simulink model "px4demo_Send_All_Data"  (R2016b)
settings: Solver=FixedStepDiscrete  StartTime=0.0  StopTime=inf  FixedStep=0.01  RelTol=1e-3  EnableMultiTasking=on
undefined symbols (not defined in the file): dt_pixhawk
libraries: pixhawk_slib_sensors_actuators x8, pixhawk_slib_ADC_serial x2
settings Model: Creator=darenlee  LastModifiedBy=ers
settings DataIOCC: LimitDataPoints=on  SaveFormat=StructureWithTime
settings OptimizationCC: DefaultParameterBehavior=Inlined  LifeSpan=1  MaxStackSize=64
settings DebuggingCC: AllowSymbolicDim=off  SFUnexpectedBacktrackingDiag=warning  SFNoUnconditionalDefaultTransitionDiag=warning  SFExecutionAtInitializationDiag=none
settings HardwareCC: ProdBitPerPointer=32  ProdBitPerSizeT=32  ProdBitPerPtrDiffT=32  ProdLargestAtomicInteger=Long  ProdLargestAtomicFloat=Double  ProdIntDivRoundTo=Undefined  ProdWordSize=32  ProdHWDeviceType=ARM Compatible->ARM Cortex
settings ModelReferenceCC: PropagateSignalLabelsOutOfModel=off
settings RTWCC: SystemTargetFile=ert.tlc  HardwareBoard=Pixhawk PX4  TLCOptions=-aInlineSetEventsForThisBaseRateFcn=TLC_FALSE -aSuppressMultiTaskScheduler=TLC_FALSE -aRateBasedStepFcn=0  TemplateMakefile=ert_default_tmf  Description=Embedded Coder  GenerateReport=on  Toolchain=Pixhawk Toolchain  IncludeHyperlinkInReport=on  LaunchReport=on  GenerateTraceInfo=on  GenerateTraceReport=on  GenerateTraceReportSl=on  GenerateTraceReportSf=on  GenerateTraceReportEml=on
settings CodeAppCC: IgnoreCustomStorageClasses=off
settings ERTTargetCC: ExtModeTransport=1  ExtModeMexFile=ext_serial_win32_comm  ExtModeMexArgs=1 8 115200  ERTCustomFileTemplate=PX4_codertarget_file_process.tlc  ConvertIfToSwitch=off  SuppressUnreachableDefaultCases=off
settings ConfigComp: CovMetricSettings=dw  CovHtmlReporting=on  CovSaveCumulativeToWorkspaceVar=on  CovSaveSingleToWorkspaceVar=on  CovExternalEMLEnable=off

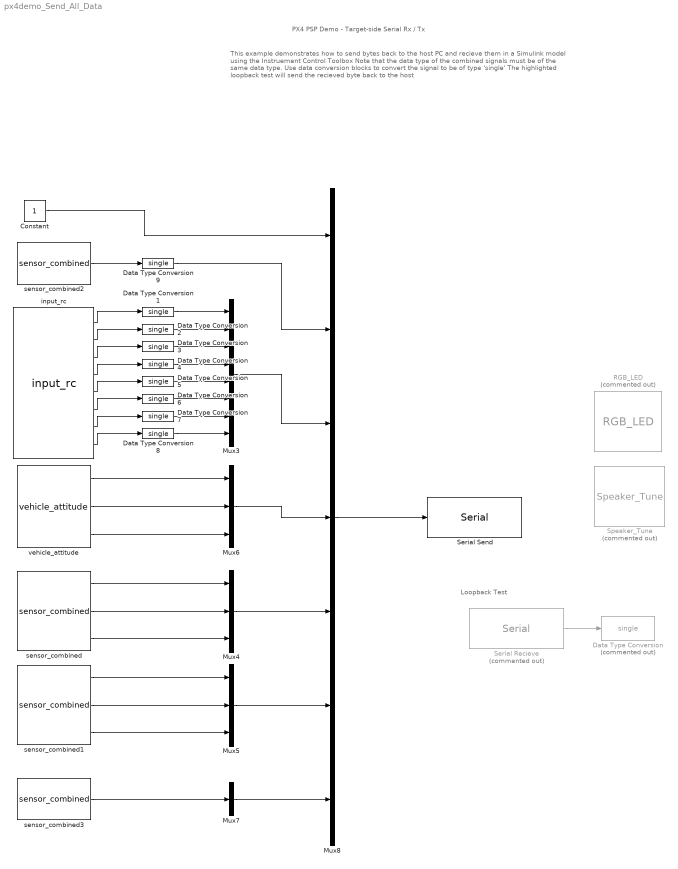
== system px4demo_Send_All_Data ==
  note: Loopback Test
  note: This example demonstrates how to send bytes back to the host PC
      | and recieve them in a Simulink model using the Instruement Control Toolbox
      |
      | Note that the data type of the combined signals must be of the same data type.
      | Use data conversion blocks to convert the signal to be of type 'single'
      |
      | The highlighted loopback test will send the recieved byte back to the host
  note: PX4 PSP Demo - Target-side Serial Rx / Tx
  Constant : Constant  OutDataTypeStr=single  SampleTime=dt_pixhawk
  Data Type Conversion : DataTypeConversion  Commented=on  OutDataTypeStr=single
  Data Type Conversion{1..9} (9 alike) : DataTypeConversion  OutDataTypeStr=single
  Mux3 : Mux  Inputs=8
  Mux4 : Mux  Inputs=3
  Mux5 : Mux  Inputs=3
  Mux6 : Mux  Inputs=3
  Mux7 : Mux  Inputs=1
  Mux8 : Mux  Inputs=7
  RGB_LED : pixhawk_slib_sensors_actuators/RGB_LED  Commented=on
  Serial Recieve : pixhawk_slib_ADC_serial/Serial  Commented=on  DeviceName=/dev/ttyS6  ReadOrWrite=Reading  BaudRateStr=115200  block=off  WriteStatus=off  Terminator=off  Header=off  NumBytesRead=1  TerminatorChar=\n  HeaderData=[ uint8( hex2dec( 'DE' ) ), uint8( hex2dec( 'AD' ) ), uint8( hex2dec( 'C0' ) ), uint8( hex2dec( 'DE' ) ) ]  SimulateUsing=Code generation
  Serial Send : pixhawk_slib_ADC_serial/Serial  DeviceName=/dev/ttyS6  ReadOrWrite=Writing  BaudRateStr=115200  block=off  WriteStatus=on  Terminator=off  Header=on  NumBytesRead=4  TerminatorChar=\n  HeaderData=[ uint8( hex2dec( '41' ) ), uint8( hex2dec( '42' ) ), uint8( hex2dec( '43' ) ), uint8( hex2dec( '41' ) ) ]  SimulateUsing=Code generation
  Speaker_Tune : pixhawk_slib_sensors_actuators/Speaker_Tune  Commented=on
  input_rc : pixhawk_slib_sensors_actuators/input_rc  sampletime=dt_pixhawk  channel1=on  channel2=on  channel3=on  channel4=on  channel5=on  channel6=on  channel7=on  channel8=on  ch_count=off  rssi=off  rc_failsafe=off  rc_lost=off  rc_inputsource=off
  sensor_combined : pixhawk_slib_sensors_actuators/sensor_combined  sampletime=dt_pixhawk  show_mag=off  show_acc=off  show_gyro=on  show_baro=off  show_ts=off
  sensor_combined1 : pixhawk_slib_sensors_actuators/sensor_combined  sampletime=dt_pixhawk  show_mag=off  show_acc=on  show_gyro=off  show_baro=off  show_ts=off
  sensor_combined2 : pixhawk_slib_sensors_actuators/sensor_combined  sampletime=dt_pixhawk  show_mag=off  show_acc=off  show_gyro=off  show_baro=off  show_ts=on
  sensor_combined3 : pixhawk_slib_sensors_actuators/sensor_combined  sampletime=dt_pixhawk  show_mag=off  show_acc=off  show_gyro=off  show_baro=on  show_ts=off
  vehicle_attitude : pixhawk_slib_sensors_actuators/vehicle_attitude  sampletime=dt_pixhawk  show_r=on  show_p=on  show_y=on  show_q=off
  wires:
  Serial Recieve/1 -> Data Type Conversion/1
  input_rc/2 -> Data Type Conversion2/1
  input_rc/3 -> Data Type Conversion3/1
  input_rc/4 -> Data Type Conversion4/1
  input_rc/5 -> Data Type Conversion5/1
  input_rc/1 -> Data Type Conversion1/1
  input_rc/6 -> Data Type Conversion6/1
  input_rc/7 -> Data Type Conversion7/1
  input_rc/8 -> Data Type Conversion8/1
  Data Type Conversion5/1 -> Mux3/5
  Data Type Conversion6/1 -> Mux3/6
  Data Type Conversion7/1 -> Mux3/7
  Data Type Conversion8/1 -> Mux3/8
  Data Type Conversion3/1 -> Mux3/3
  Data Type Conversion4/1 -> Mux3/4
  Data Type Conversion2/1 -> Mux3/2
  Data Type Conversion1/1 -> Mux3/1
  vehicle_attitude/2 -> Mux6/2
  vehicle_attitude/3 -> Mux6/3
  vehicle_attitude/1 -> Mux6/1
  Constant/1 -> Mux8/1
  Mux3/1 -> Mux8/3
  Mux6/1 -> Mux8/4
  Mux5/1 -> Mux8/6
  Mux7/1 -> Mux8/7
  Mux8/1 -> Serial Send/1
  Mux4/1 -> Mux8/5
  sensor_combined/1 -> Mux4/1
  sensor_combined/2 -> Mux4/2
  sensor_combined/3 -> Mux4/3
  sensor_combined1/1 -> Mux5/1
  sensor_combined1/2 -> Mux5/2
  sensor_combined1/3 -> Mux5/3
  sensor_combined3/1 -> Mux7/1
  sensor_combined2/1 -> Data Type Conversion9/1
  Data Type Conversion9/1 -> Mux8/2
